simulink library "relay_modbus_lib"  (Simulink 8.1)
settings: Solver=ode45  StartTime=0.0  StopTime=10.0  RelTol=1e-3
undefined symbols (not defined in the file): relay_par, Ts
libraries: powerlib_extras x3, relay_PLL_lib x2, simulink x2, relay_PQSPF_lib x1, relay_ANSI_F25_lib x1, relay_mgc_cmd_lib x1, relay_tripOutMng_lib x1, relay_ANSI_functions_lib x1
settings Model: Creator=RE25624  LastModifiedBy=re25624

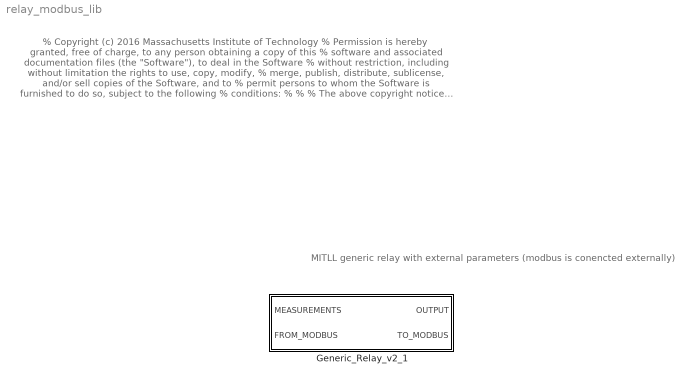
== system relay_modbus_lib ==
  note: MITLL generic relay with external parameters (modbus is conencted externally)
  note: % Copyright (c) 2016 Massachusetts Institute of Technology
      | % Permission is hereby granted, free of charge, to any person obtaining a copy of this
      | % software and associated documentation files (the "Software"), to deal in the Software
      | % without restriction, including without limitation the rights to use, copy, modify,
      | % merge, publish, distribute, sublicense, and/or sell copies of the Software, and to
      | % permit persons to whom the Software is furnished to do so, subject to the following
      | % conditions:
      | %
      | %
      | % The above copyright notice and this permission notice shall be included in
      | % all copies or substantial portions of the Software.
      | %
      | % THE SOFTWARE IS PROVIDED "AS IS", WITHOUT WARRANTY OF ANY KIND, EXPRESS OR IMPLIED,
      | % INCLUDING BUT NOT LIMITED TO THE WARRANTIES OF MERCHANTABILITY, FITNESS FOR A
      | % PARTICULAR PURPOSE AND NONINFRINGEMENT. IN NO EVENT SHALL THE AUTHORS OR COPYRIGHT
      | % HOLDERS BE LIABLE FOR ANY CLAIM, DAMAGES OR OTHER LIABILITY, WHETHER IN AN ACTION
      | % OF CONTRACT, TORT OR OTHERWISE, ARISING FROM, OUT OF OR IN CONNECTION WITH THE
      | % SOFTWARE OR THE USE OR OTHER DEALINGS IN THE SOFTWARE.
      | %
      | %
      | %%
  Generic_Relay_v2_1 : Subsystem  mask(Generic Relay){Ts=Ts, relay_settings=[relay_par(2,:)]}
      mask prompts: Ts "Sampling Time [Sec]"; relay_settings "Relay Settings"
      mask help:
      | This relay simulates functions: synchronizing or synchronism-check (25), phase instantaneous overcurrent (50P), AC inverse time overcurrent (51P), undervoltage relay (27), and overvoltage relay (59).
      |
      | FEATURES:
      | 1) Receives commands from the microgrid controller via MODBUS/TCP
      | 2) Two groups of interchangeable protection settings
      |     - To be used for grid-tied and islanded protection modes
      | 3) Locked-out only enabled for functions (50P), (51P)
      |     - (27) and (59) pickups will be model inputs for the next revision
      | 4) MODBUS commands expected in the following order:
      |    a) Functions reset (Holding Reg# 2000)
      |    b) Breaker state   (Holding Reg# 2001)
      |    c) Protection mode (Holding Reg# 2002)
      |       - bit = 0; parameter group#1 (default)
      |       - bit = 1; parameter group#2
      |
      | See help or integration packet for further information.
      mask Help:
      | Procedure to reclose a breaker:
      | 1) reset all functions (Holding Reg# 2000)
      | 2) set breaker state (Holding Reg# 2001) to generate a close signal
      | 	- Synch-check (25) will automatically activate
      | 	- bit = 0, trip functions are active
      | 	- bit = 1, trip functions are not active
      | 
      | 
      | 
      | Field format/order for relay settings:
      | 	- Assuming zero delay between group settings changes
      | 
      | 1.  Relay#
      | 2.  Nominal VRMSLL
      | 3.  Max. Slip Voltage [%]
      | 4.  Max. Slip Angle [degree]
      | 5.  Max. Slip Frequency [Hz]
      | 6.  27P and 59P Trip Delay [Sec]
      | 7.  CT Primary
      | 
      | Parameter Group #1
      | 8.  50P Instantaneous overcurrent (IOC) Trip Pickup
      | 9.  50P IOC Trip Delay [sec]
      | 10.  51P Time overcurrent (TOC) Trip Pickup
      | 11.  51P Curve Type
      | 12.  51P TOC Time Dial
      | 13.  27P Trip Pickup [pu]
      | 14.  59P Trip Pickup [pu]
      | 
      | Parameter Group #2
      | 15.  50P IOC Trip Pickup
      | 16.  50P IOC Trip Delay [sec]
      | 17.  51P TOC Trip Pickup
      | 18.  51P Curve Type
      | 19.  51P TOC Time Dial
      | 20.  27P Trip Pickup [pu]
      | 21.  59P Trip Pickup [pu]
      | 
      | Available TCC Characteristics:
      | 	- The degree of inverseness for each curve approximates SEL-751
      | 
      | 51P Curve
      | 1: moderate inverse
      | 2: inverse
      | 3: very inverse
      | 4: extremely inverse
      | 
      | References:
      | [1] IEEE Std. C37.112-1996
      | [2] SEL 751 Instruction manual
      | [3] MIT-LL 2nd Microgrid Controller Symposium - Integration Packet

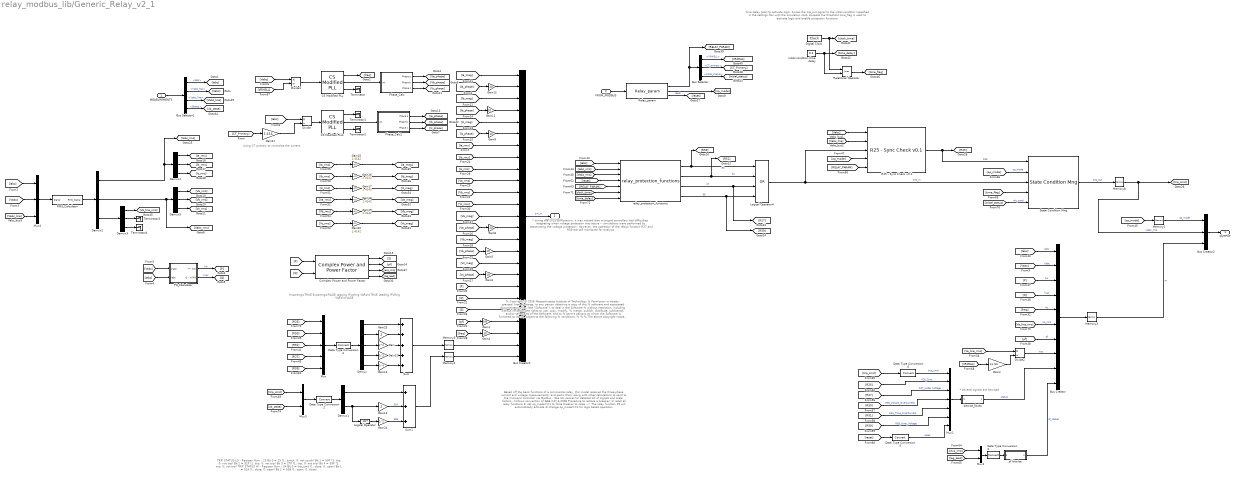
== system relay_modbus_lib/Generic_Relay_v2_1 ==
  note: % Copyright (c) 2016 Massachusetts Institute of Technology
      | % Permission is hereby granted, free of charge, to any person obtaining a copy of this
      | % software and associated documentation files (the "Software"), to deal in the Software
      | % without restriction, including without limitation the rights to use, copy, modify,
      | % merge, publish, distribute, sublicense, and/or sell copies of the Software, and to
      | % permit persons to whom the Software is furnished to do so, subject to the following
      | % conditions:
      | %
      | %
      | % The above copyright notice and this permission notice shall be included in
      | % all copies or substantial portions of the Software.
      | %
      | % THE SOFTWARE IS PROVIDED "AS IS", WITHOUT WARRANTY OF ANY KIND, EXPRESS OR IMPLIED,
      | % INCLUDING BUT NOT LIMITED TO THE WARRANTIES OF MERCHANTABILITY, FITNESS FOR A
      | % PARTICULAR PURPOSE AND NONINFRINGEMENT. IN NO EVENT SHALL THE AUTHORS OR COPYRIGHT
      | % HOLDERS BE LIABLE FOR ANY CLAIM, DAMAGES OR OTHER LIABILITY, WHETHER IN AN ACTION
      | % OF CONTRACT, TORT OR OTHERWISE, ARISING FROM, OUT OF OR IN CONNECTION WITH THE
      | % SOFTWARE OR THE USE OR OTHER DEALINGS IN THE SOFTWARE.
      | %
      | %
      | %%
  note: * during the 2015 sympoaium, it was noticed that microgrid controllers had
      | difficulties integrating when voltage protection was active
      |
      | -- simulations were performed by deactivating the voltage protection.
      | However, the operation of the relays function  R27 and R59 are still monitored for analysis
  note: Importing=TRUE
      | Exporting=FALSE
      |
      | Lagging (Pushing VARs)=TRUE
      | Leading (Pulling VARs)=FALSE
  note: * several signals are bitwised
  note: Using CT primary to normalize the current.
  note: TRIP STATUS LO - Register Num.: 23
      | Bit 0 = 25  (1: synch, 0: not synch)
      | Bit 1 = 50P (1: trip, 0: not trip)
      | Bit 2 = 51P (1: trip, 0: not trip)
      | Bit 3 = 27P (1: trip, 0: not trip)
      | Bit 4 = 59P (1: trip, 0: not trip)
      |
      | TRIP STATUS HI - Register Num.: 24
      | Bit 0 = trip_cmd  (1: close, 0: open)
      | Bit 1 = 52A (1: close, 0: open)
      | Bit 2 = 52B (1: open, 0: close)
  note: Based off the basic functions of a commercial relay, this model receives
      | the three-phase current and voltage measurements, and packs
      | them along with other calculations to send to the microgrid
      | controller via Modbus
      |
      | - See HIL packet for detailed list of signals and scale factors
      | - Follows convention of IEEE C37.2-2008
      |
      | Procedure to reclose a breaker:
      | 1) reset all relay functions
      | 2) set op_mode==1 to force breaker to close
      |    --> The relay function 25 will automatically activate
      | 3) change op_mode==0 for logic based operation
  note: time delay [sec] to activate logic. Forces the trip_out signal to the initial condition
      | (specified in the settings file) until the simulation clock exceeds the threshold
      |
      | time_flag is used to activate logic and enable protection functions
  MEASUREMENTS : Inport
  FROM_MODBUS : Inport  Port=2
  Bus Creator : BusCreator  Inputs=10
  Bus Creator1 : BusCreator  Inputs=25
  Bus Creator2 : BusCreator  Inputs=3
  Bus Selector : BusSelector  OutputSignals=VRMSLL,CT_primary,Initial_status
  Bus Selector1 : BusSelector  OutputSignals=Iabc,Vabc_bus,Vabc_line,Status
  CS Modified PLL : relay_PLL_lib/CS Modified PLL  Fmin=50  Par_Init=[0 60]  ParK=[ 180 3200 1 ]  Ts=Ts  AGC=off
  CS Modified PLL1 : relay_PLL_lib/CS Modified PLL  Fmin=50  Par_Init=[0 60]  ParK=[ 180 3200 1 ]  Ts=Ts  AGC=off
  Complex Power and Power Factor : relay_PQSPF_lib/Complex Power and Power Factor
  Data Type Conversion{2..6} (5 alike) : DataTypeConversion
  Demux : Demux  Outputs=5
  Demux1 : Demux  Outputs=2
  Demux2 : Demux  Outputs=[3 3 3]
  Demux3 : Demux  Outputs=3
  Demux4 : Demux  Outputs=3
  Demux5 : Demux  Outputs=3
  Digital Clock : DigitalClock  SampleTime=Ts
  Divide : Product  Inputs=*/
  Divide1 : Product  Inputs=*/
  Divide2 : Product  Inputs=*/
  Gain : Gain  Gain=2^2
  Gain1 : Gain  Gain=100
  Gain{3..5,8..9,11..12} (7 alike) : Gain  Gain=10
  Gain13 : Gain  Gain=2
  Gain14 : Gain  Gain=2^4
  Gain{15..20} (6 alike) : Gain  Gain=1.4142
  Gain2 : Gain  Gain=1/1.732
  Gain21 : Gain  Gain=1.414
  Gain22 : Gain  Gain=2^3
  Gain23 : Gain  Gain=2
  Gain24 : Gain  Gain=2^2
  Logical Operator : Logic  Operator=NOT  AllPortsSameDT=off  OutDataTypeStr=boolean
  Logical Operator4 : Logic  Operator=OR  Inputs=4  AllPortsSameDT=off  OutDataTypeStr=boolean
  Memory{1..3,8..9} (5 alike) : Memory
  Mux : Mux  Inputs=5
  Mux1 : Mux  Inputs=7
  Mux2 : Mux  Inputs=2
  Mux3 : Mux  Inputs=2
  Mux4 : Mux  Inputs=3
  PQ_Calculator : Subsystem
  Phase_Calc : Subsystem
  Phase_Calc1 : Subsystem
  R25 - Sync Check v0.1 : relay_ANSI_F25_lib/R25 - Sync Check v0.1  Ts=Ts
  RMS_Calculator : Subsystem
  Relational Operator : RelationalOperator  OutDataTypeStr=boolean
  Relay_param : relay_mgc_cmd_lib/Relay_param  relay_settings=relay_settings
  State Condition Mng : relay_tripOutMng_lib/State Condition Mng
  Sum : Sum  Inputs=+++++
  Sum1 : Sum  Inputs=+++
  Terminator{,1..4} (5 alike) : Terminator
  bitwise_faults : Subsystem
  initial condition time delay : Constant  Value=0.2
  pf bitwise : Subsystem
  relay_protection_functions : relay_ANSI_functions_lib/relay_protection_functions  Ts=Ts
  OUTPUT : Outport
  TO_MODBUS : Outport  Port=2
  wires:
  Relational Operator/1 -> [time_flag]
  Demux3/3 -> Terminator4/1
  Demux3/2 -> Terminator3/1
  Demux2/3 -> Demux3/1
  Demux3/1 -> [Va_line_rms]
  RMS_Calculator/1(RMS_Signal) -> Demux2/1
  Mux4/1 -> RMS_Calculator/1(Signal)
  [Vabc_line] -> Mux4/3
  Gain2/1 -> Divide2/2
  Logical Operator/1 -> Gain24/1
  [Initial_status] -> State Condition Mng/5  "init_cond"
  Bus Selector/3 -> [Initial_status]  "<Initial_status>"
  [time_delay] -> relay_protection_functions/7
  [clock_time] -> relay_protection_functions/6
  Relay_param/3 -> [reset]  "reset"
  initial condition time delay/1 -> [time_delay], Relational Operator/2
  [time_flag] -> State Condition Mng/4
  Digital Clock/1 -> [clock_time], Relational Operator/1
  Gain21/1 -> Divide/2
  Relay_param/2 -> [op_mode]
  [Va_line_rms] -> Divide2/1
  [VRMSLL] -> Gain2/1
  [VRMSLL] -> Divide1/2
  Divide1/1 -> CS Modified PLL/1
  [Vabc] -> Divide1/1
  Bus Selector/1 -> [VRMSLL]  "<VRMSLL>"
  [RELAY_PARAM] -> R25 - Sync Check v0.1/5
  [RELAY_PARAM] -> relay_protection_functions/5
  [Iabc] -> relay_protection_functions/1
  [Vabc_rms] -> relay_protection_functions/3
  [Iabc_rms] -> relay_protection_functions/2
  [reset] -> relay_protection_functions/4
  Relay_param/1 -> Bus Selector/1, [RELAY_PARAM]
  Bus Selector/2 -> [CT_Primary]  "<CT_primary>"
  Data Type Conversion3/1 -> pf bitwise/1(S)
  Memory3/1 -> Bus Creator2/3  "m"
  [lag_lead] -> Mux2/2
  [exp_imp] -> Mux2/1
  pf bitwise/1(s) -> Bus Creator/10  "pf_states"
  Mux2/1 -> Data Type Conversion3/1
  Complex Power and Power Factor/4 -> [lag_lead]
  Complex Power and Power Factor/3 -> [exp_imp]
  Complex Power and Power Factor/2 -> [pf]
  Complex Power and Power Factor/1 -> [S]
  [Q] -> Complex Power and Power Factor/2
  [P] -> Complex Power and Power Factor/1
  Bus Creator2/1 -> OUTPUT/1
  Memory1/1 -> Bus Creator2/1  "op_mode"
  Bus Creator/1 -> Memory3/1
  MEASUREMENTS/1 -> Bus Selector1/1
  Bus Selector1/3 -> [Vabc_line]  "<Vabc_line>"
  Bus Selector1/2 -> [Vabc]  "<Vabc_bus>"
  Bus Selector1/1 -> [Iabc]  "<Iabc>"
  [Vabc_line] -> R25 - Sync Check v0.1/2
  Data Type Conversion6/1 -> Mux1/1  "trip_cmd"
  Data Type Conversion5/1 -> Mux1/7  "reset"
  [R59] -> Mux1/6  "R59_Over_Voltage"
  [R51] -> Mux1/5  "R51_Time_OverCurrent"
  [R50] -> Mux1/4  "R50_Instant_OverCurrent"
  [R27] -> Mux1/3  "R27_Under Voltage"
  [R25] -> Mux1/2  "R25_Sync"
  [trip_cmd] -> Data Type Conversion6/1
  [reset] -> Data Type Conversion5/1
  bitwise_faults/1(s) -> Bus Creator/9  "status"
  Mux1/1 -> bitwise_faults/1(S)
  relay_protection_functions/4 -> [R59], Logical Operator4/4  "59"
  relay_protection_functions/3 -> [R27], Logical Operator4/3  "27"
  Divide2/1 -> Bus Creator/8  "Vpu"
  Gain15/1 -> [Ia_mag]
  Gain16/1 -> [Ib_mag]
  Gain17/1 -> [Ic_mag]
  Gain18/1 -> [Va_mag]
  Gain19/1 -> [Vb_mag]
  Gain20/1 -> [Vc_mag]
  [Vc_rms] -> Gain20/1
  [Vb_rms] -> Gain19/1
  [Va_rms] -> Gain18/1
  [Ic_rms] -> Gain17/1
  [Ib_rms] -> Gain16/1
  [Ia_rms] -> Gain15/1
  [Vabc] -> R25 - Sync Check v0.1/1
  Gain4/1 -> Bus Creator1/23
  Gain1/1 -> Bus Creator1/22
  [S] -> Bus Creator1/21
  [Q] -> Bus Creator1/20
  [P] -> Bus Creator1/19
  Gain3/1 -> Bus Creator1/18
  [Vc_mag] -> Bus Creator1/17
  Gain5/1 -> Bus Creator1/16
  [Vb_mag] -> Bus Creator1/15
  Gain8/1 -> Bus Creator1/14
  [Va_mag] -> Bus Creator1/13
  [Vc_rms] -> Bus Creator1/12
  [Vb_rms] -> Bus Creator1/11
  [Va_rms] -> Bus Creator1/10
  [Ic_rms] -> Bus Creator1/9
  [Ib_rms] -> Bus Creator1/8
  [Ia_rms] -> Bus Creator1/7
  Gain9/1 -> Bus Creator1/6
  [Ic_mag] -> Bus Creator1/5
  Gain11/1 -> Bus Creator1/4
  [Ib_mag] -> Bus Creator1/3
  Gain12/1 -> Bus Creator1/2
  [Ia_mag] -> Bus Creator1/1
  [pf] -> Bus Creator/7  "pf"
  [Va_line_rms] -> Bus Creator/6  "Va_rms"
  [freq] -> Bus Creator/5  "Hz"
  CS Modified PLL/3 -> Terminator/1
  CS Modified PLL1/3 -> Terminator2/1
  CS Modified PLL1/1 -> Terminator1/1
  CS Modified PLL/2 -> Phase_Calc/1(wt)
  CS Modified PLL/1 -> [freq]
  CS Modified PLL1/2 -> Phase_Calc1/1(wt)
  [op_mode] -> R25 - Sync Check v0.1/4
  Logical Operator4/1 -> State Condition Mng/3, R25 - Sync Check v0.1/3  "trip_in"
  [op_mode] -> State Condition Mng/2  "op_mode"
  R25 - Sync Check v0.1/1 -> State Condition Mng/1, [R25]  "R25"
  Memory8/1 -> Bus Creator2/2, [trip_cmd]  "Logic_trip"
  [op_mode] -> Memory1/1
  Memory2/1 -> Bus Creator1/25
  Memory9/1 -> Bus Creator1/24
  Data Type Conversion4/1 -> Demux/1
  Demux/1 -> Sum/1
  Mux/1 -> Data Type Conversion4/1
  relay_protection_functions/2 -> [R51], Logical Operator4/2  "51"
  Sum/1 -> Memory9/1
  Sum1/1 -> Memory2/1
  relay_protection_functions/1 -> [R50], Logical Operator4/1  "50"
  [Ia_phase] -> Gain12/1
  [Ib_phase] -> Gain11/1
  [Ic_phase] -> Gain9/1
  [Va_phase] -> Gain8/1
  [Vb_phase] -> Gain5/1
  [Vc_phase] -> Gain3/1
  [CT_Primary] -> Gain21/1
  Divide/1 -> CS Modified PLL1/1
  Phase_Calc1/3(Phase c) -> [Ic_phase]
  Phase_Calc1/2(Phase b) -> [Ib_phase]
  Phase_Calc1/1(Phase a) -> [Ia_phase]
  [Iabc] -> Divide/1
  Phase_Calc/3(Phase c) -> [Vc_phase]
  Phase_Calc/2(Phase b) -> [Vb_phase]
  Phase_Calc/1(Phase a) -> [Va_phase]
  [Q] -> Bus Creator/4  "kvar"
  [P] -> Bus Creator/3  "kw"
  [pf] -> Gain1/1
  [freq] -> Gain4/1
  Bus Creator1/1 -> TO_MODBUS/1  "sm_in"
  FROM_MODBUS/1 -> Relay_param/1
  [Vabc] -> Bus Creator/2  "Vabc"
  [Iabc] -> Bus Creator/1  "Iabc"
  [Vabc] -> PQ_Calculator/1(Vabc)
  [Iabc] -> PQ_Calculator/2(Iabc)
  PQ_Calculator/1(P - kW) -> [P]  "kw"
  PQ_Calculator/2(Q - kVAR) -> [Q]  "kvar"
  [Iabc] -> Mux4/1
  [Vabc] -> Mux4/2
  Demux2/1 -> Demux4/1, [Iabc_rms]
  Demux2/2 -> Demux5/1, [Vabc_rms]
  Demux4/3 -> [Ic_rms]
  Demux4/2 -> [Ib_rms]
  Demux4/1 -> [Ia_rms]
  Demux5/1 -> [Va_rms]
  Demux5/2 -> [Vb_rms]
  Demux5/3 -> [Vc_rms]
  State Condition Mng/1 -> Memory8/1  "trip_out"
  Bus Selector1/4 -> [cb_state]  "<Status>"
  [R25] -> Mux/1
  [R50] -> Mux/2
  [R51] -> Mux/3
  [R27] -> Mux/4
  [R59] -> Mux/5
  Demux/2 -> Gain23/1
  Demux/3 -> Gain/1
  Demux/4 -> Gain22/1
  Gain23/1 -> Sum/2
  Gain/1 -> Sum/3
  Gain22/1 -> Sum/4
  Mux3/1 -> Data Type Conversion2/1
  Gain13/1 -> Sum1/2  "52A"
  Demux1/1 -> Sum1/1
  Data Type Conversion2/1 -> Demux1/1
  Gain14/1 -> Sum/5
  Demux/5 -> Gain14/1
  [trip_cmd] -> Mux3/1
  [cb_state] -> Mux3/2
  Gain24/1 -> Sum1/3  "52B"
  Demux1/2 -> Logical Operator/1, Gain13/1

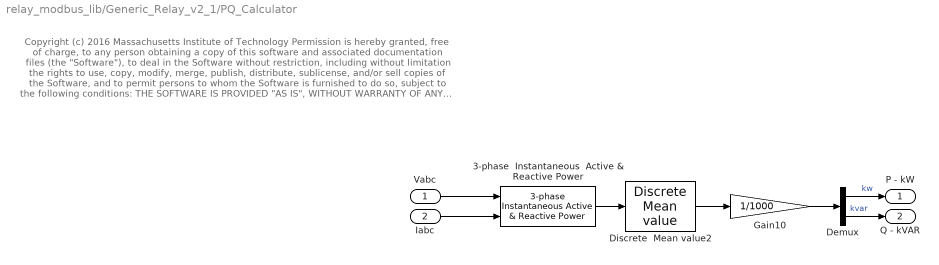
== system relay_modbus_lib/Generic_Relay_v2_1/PQ_Calculator ==
  note: Copyright (c) 2016 Massachusetts Institute of Technology
      | Permission is hereby granted, free of charge, to any person obtaining a copy of this software and associated documentation files (the "Software"), to deal
      | in the Software without restriction, including without limitation the rights to use, copy, modify, merge, publish, distribute, sublicense, and/or sell copies of the
      | Software, and to permit persons to whom the Software is furnished to do so, subject to the following conditions:
      |
      | THE SOFTWARE IS PROVIDED "AS IS", WITHOUT WARRANTY OF ANY KIND, EXPRESS OR IMPLIED, INCLUDING BUT NOT LIMITED TO THE
      | WARRANTIES OF MERCHANTABILITY, FITNESS FOR A PARTICULAR PURPOSE AND NONINFRINGEMENT. IN NO EVENT SHALL THE AUTHORS
      | OR COPYRIGHT HOLDERS BE LIABLE FOR ANY CLAIM, DAMAGES OR OTHER LIABILITY, WHETHER IN AN ACTION OF CONTRACT, TORT OR
      | OTHERWISE, ARISING FROM, OUT OF OR IN CONNECTION WITH THE SOFTWARE OR THE USE OR OTHER DEALINGS IN THE SOFTWARE
  Vabc : Inport
  Iabc : Inport  Port=2
  3-phase  Instantaneous  Active & Reactive Power : powerlib_extras/Measurements/3-phase  Instantaneous  Active & Reactive Power
  Demux : Demux  Outputs=2
  Discrete  Mean value2 : powerlib_extras/Discrete Measurements/Discrete  Mean value  Freq=60  Vinit=0  Ts=Ts
  Gain10 : Gain  Gain=1/1000
  P - kW : Outport
  Q - kVAR : Outport  Port=2
  wires:
  Gain10/1 -> Demux/1
  3-phase  Instantaneous  Active & Reactive Power/1 -> Discrete  Mean value2/1
  Discrete  Mean value2/1 -> Gain10/1
  Vabc/1 -> 3-phase  Instantaneous  Active & Reactive Power/1
  Iabc/1 -> 3-phase  Instantaneous  Active & Reactive Power/2
  Demux/1 -> P - kW/1  "kw"
  Demux/2 -> Q - kVAR/1  "kvar"

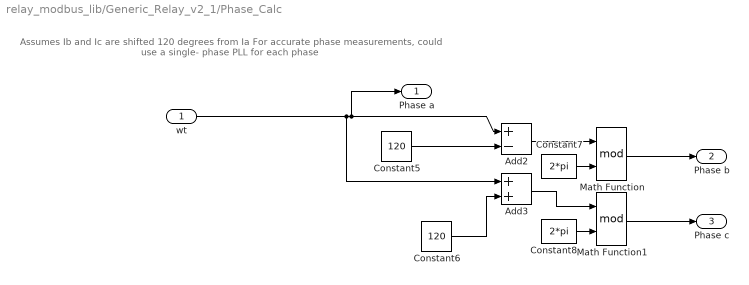
== system relay_modbus_lib/Generic_Relay_v2_1/Phase_Calc ==
  note: Assumes Ib and Ic are shifted 120 degrees from Ia
      | For accurate phase measurements, could use a single-
      | phase PLL for each phase
  wt : Inport
  Add2 : Sum  Inputs=+-
  Add3 : Sum
  Constant5 : Constant  Value=120
  Constant6 : Constant  Value=120
  Constant7 : Constant  Value=2*pi
  Constant8 : Constant  Value=2*pi
  Math Function : Math  Operator=mod  SaturateOnIntegerOverflow=on
  Math Function1 : Math  Operator=mod  SaturateOnIntegerOverflow=on
  Phase a : Outport
  Phase b : Outport  Port=2
  Phase c : Outport  Port=3
  wires:
  Math Function1/1 -> Phase c/1
  Math Function/1 -> Phase b/1
  Constant8/1 -> Math Function1/2
  Add3/1 -> Math Function1/1
  Add2/1 -> Math Function/1
  Constant7/1 -> Math Function/2
  wt/1 -> Add3/1, Phase a/1, Add2/1
  Constant6/1 -> Add3/2
  Constant5/1 -> Add2/2

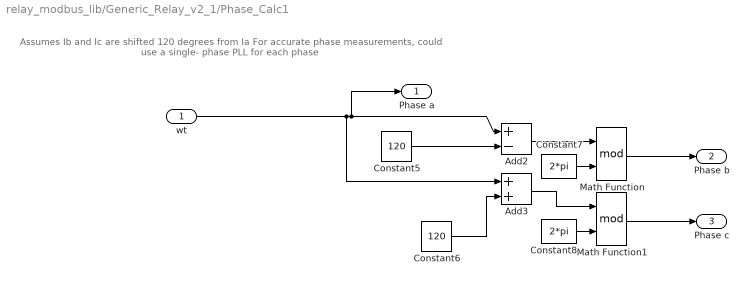
== system relay_modbus_lib/Generic_Relay_v2_1/Phase_Calc1 ==
  note: Assumes Ib and Ic are shifted 120 degrees from Ia
      | For accurate phase measurements, could use a single-
      | phase PLL for each phase
  wt : Inport
  Add2 : Sum  Inputs=+-
  Add3 : Sum
  Constant5 : Constant  Value=120
  Constant6 : Constant  Value=120
  Constant7 : Constant  Value=2*pi
  Constant8 : Constant  Value=2*pi
  Math Function : Math  Operator=mod  SaturateOnIntegerOverflow=on
  Math Function1 : Math  Operator=mod  SaturateOnIntegerOverflow=on
  Phase a : Outport
  Phase b : Outport  Port=2
  Phase c : Outport  Port=3
  wires:
  Constant5/1 -> Add2/2
  Constant6/1 -> Add3/2
  wt/1 -> Add2/1, Phase a/1, Add3/1
  Constant7/1 -> Math Function/2
  Add2/1 -> Math Function/1
  Add3/1 -> Math Function1/1
  Constant8/1 -> Math Function1/2
  Math Function/1 -> Phase b/1
  Math Function1/1 -> Phase c/1

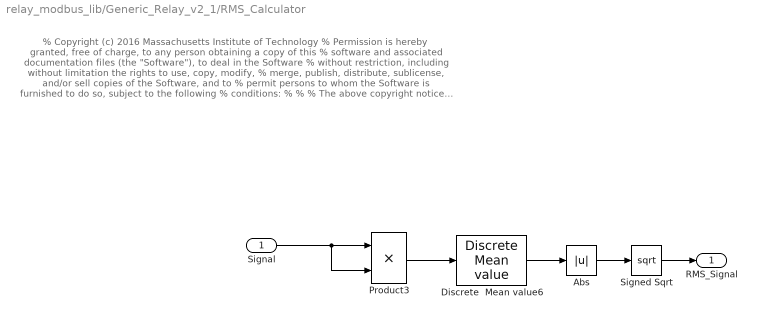
== system relay_modbus_lib/Generic_Relay_v2_1/RMS_Calculator ==
  note: % Copyright (c) 2016 Massachusetts Institute of Technology
      | % Permission is hereby granted, free of charge, to any person obtaining a copy of this
      | % software and associated documentation files (the "Software"), to deal in the Software
      | % without restriction, including without limitation the rights to use, copy, modify,
      | % merge, publish, distribute, sublicense, and/or sell copies of the Software, and to
      | % permit persons to whom the Software is furnished to do so, subject to the following
      | % conditions:
      | %
      | %
      | % The above copyright notice and this permission notice shall be included in
      | % all copies or substantial portions of the Software.
      | %
      | % THE SOFTWARE IS PROVIDED "AS IS", WITHOUT WARRANTY OF ANY KIND, EXPRESS OR IMPLIED,
      | % INCLUDING BUT NOT LIMITED TO THE WARRANTIES OF MERCHANTABILITY, FITNESS FOR A
      | % PARTICULAR PURPOSE AND NONINFRINGEMENT. IN NO EVENT SHALL THE AUTHORS OR COPYRIGHT
      | % HOLDERS BE LIABLE FOR ANY CLAIM, DAMAGES OR OTHER LIABILITY, WHETHER IN AN ACTION
      | % OF CONTRACT, TORT OR OTHERWISE, ARISING FROM, OUT OF OR IN CONNECTION WITH THE
      | % SOFTWARE OR THE USE OR OTHER DEALINGS IN THE SOFTWARE.
      | %
      | %
      | %%
  Signal : Inport
  Abs : Abs
  Discrete  Mean value6 : powerlib_extras/Discrete Measurements/Discrete  Mean value  Freq=60  Vinit=0  Ts=Ts
  Product3 : Product  RndMeth=Zero
  Signed Sqrt : Sqrt  SaturateOnIntegerOverflow=on
  RMS_Signal : Outport
  wires:
  Abs/1 -> Signed Sqrt/1
  Product3/1 -> Discrete  Mean value6/1
  Signal/1 -> Product3/1, Product3/2
  Discrete  Mean value6/1 -> Abs/1
  Signed Sqrt/1 -> RMS_Signal/1

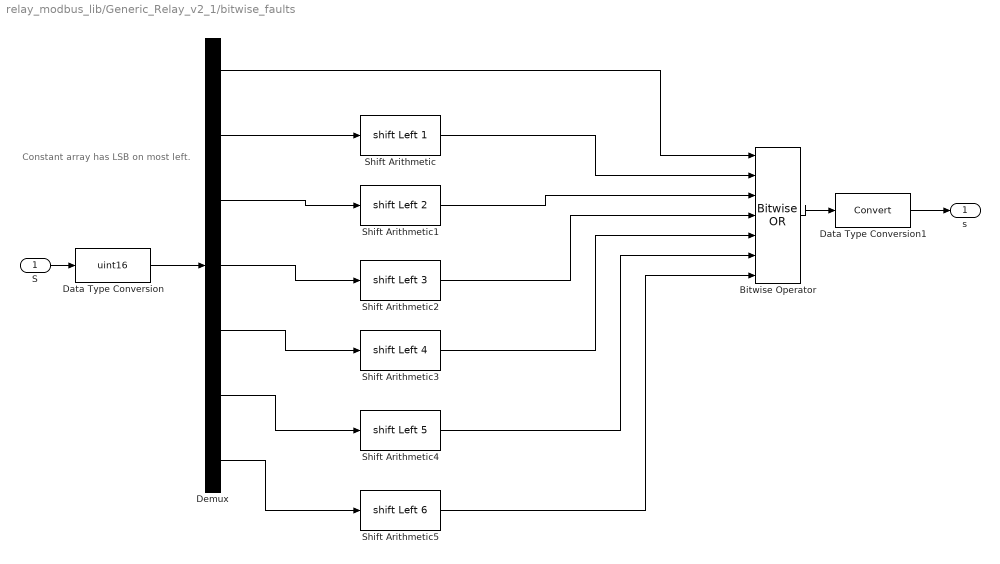
== system relay_modbus_lib/Generic_Relay_v2_1/bitwise_faults ==
  note: Constant array has LSB on most left.
  S : Inport
  Bitwise Operator : simulink/Logic and Bit Operations/Bitwise Operator  logicop=OR  UseBitMask=off  NumInputPorts=7  BitMask=bin2dec('11011001')  BitMaskRealWorld=Stored Integer
  Data Type Conversion : DataTypeConversion  OutDataTypeStr=uint16
  Data Type Conversion1 : DataTypeConversion
  Demux : Demux  Outputs=7
  Shift Arithmetic : ArithShift  BitShiftNumber=1  BitShiftDirection=Left
  Shift Arithmetic1 : ArithShift  BitShiftNumber=2  BitShiftDirection=Left
  Shift Arithmetic2 : ArithShift  BitShiftNumber=3  BitShiftDirection=Left
  Shift Arithmetic3 : ArithShift  BitShiftNumber=4  BitShiftDirection=Left
  Shift Arithmetic4 : ArithShift  BitShiftNumber=5  BitShiftDirection=Left
  Shift Arithmetic5 : ArithShift  BitShiftNumber=6  BitShiftDirection=Left
  s : Outport
  wires:
  Shift Arithmetic5/1 -> Bitwise Operator/7
  Shift Arithmetic4/1 -> Bitwise Operator/6
  Shift Arithmetic3/1 -> Bitwise Operator/5
  Shift Arithmetic2/1 -> Bitwise Operator/4
  Shift Arithmetic1/1 -> Bitwise Operator/3
  Shift Arithmetic/1 -> Bitwise Operator/2
  Demux/7 -> Shift Arithmetic5/1
  Demux/6 -> Shift Arithmetic4/1
  Demux/5 -> Shift Arithmetic3/1
  Demux/4 -> Shift Arithmetic2/1
  Demux/3 -> Shift Arithmetic1/1
  Demux/2 -> Shift Arithmetic/1
  Demux/1 -> Bitwise Operator/1
  Data Type Conversion1/1 -> s/1
  Bitwise Operator/1 -> Data Type Conversion1/1
  S/1 -> Data Type Conversion/1
  Data Type Conversion/1 -> Demux/1

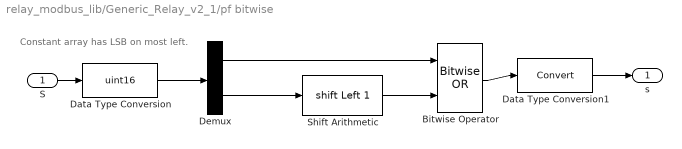
== system relay_modbus_lib/Generic_Relay_v2_1/pf bitwise ==
  note: Constant array has LSB on most left.
  S : Inport
  Bitwise Operator : simulink/Logic and Bit Operations/Bitwise Operator  logicop=OR  UseBitMask=off  NumInputPorts=2  BitMask=bin2dec('11011001')  BitMaskRealWorld=Stored Integer
  Data Type Conversion : DataTypeConversion  OutDataTypeStr=uint16
  Data Type Conversion1 : DataTypeConversion
  Demux : Demux  Outputs=2
  Shift Arithmetic : ArithShift  BitShiftNumber=1  BitShiftDirection=Left
  s : Outport
  wires:
  Data Type Conversion/1 -> Demux/1
  S/1 -> Data Type Conversion/1
  Bitwise Operator/1 -> Data Type Conversion1/1
  Data Type Conversion1/1 -> s/1
  Demux/1 -> Bitwise Operator/1
  Demux/2 -> Shift Arithmetic/1
  Shift Arithmetic/1 -> Bitwise Operator/2
